simulink model "DC_Motor_Load_PID_tuning_unit_response"  (R2015a)
settings: Solver=ode45  StartTime=0.0  StopTime=10.0  RelTol=1e-3
values from neighbouring files (symbols this model uses):
  BL = B_roller + B_material    (= 0)    [dc_motor_show_data_last.m]    (also in dc_motor_show_data_last_pos.m)
  Bm = 0.0158    [dc_motor_show_data_last.m]    (also in dc_motor_show_data_last_pos.m = 0.00093)
  JL = J_roller + J_material    (= 0.000102958)    [dc_motor_show_data_last.m]    (also in dc_motor_show_data_last_pos.m)
  Jm = 0.00252    [dc_motor_show_data_last.m]    (also in dc_motor_show_data_last_pos.m = 5.26e-05)
  Kd = Kp*Td    (= 8.33268608414)    [ZIEGLER_NICHOLCUS_METHOD_tuning_pid.m]    (also in dc_motor_show_data.m = 0.0189; dc_motor_show_data_PID_range_errors_show.m = 0.09; dc_motor_show_data_PID_range_response.m = 0.09; dc_motor_show_data_PID_test_ST.m = 0.09)
  Ke = 0.1    [DC_MOTOR.m]    (also in ZIEGLER_NICHOLCUS_METHOD_tuning_pid.m = 0.57; dc_motor_show_data.m = 0.57; dc_motor_show_data_PID_range_errors_show.m; dc_motor_show_data_PID_range_response.m)
  Ki = Kp/Ti    (= 21.5184713376)    [ZIEGLER_NICHOLCUS_METHOD_tuning_pid.m]    (also in dc_motor_show_data.m = 39.9; dc_motor_show_data_PID_range_errors_show.m = 2.98; dc_motor_show_data_PID_range_response.m = 2.98; dc_motor_show_data_PID_test_ST.m = 2.98)
  Kp = 0.2*K_cr    (= 16.4)    [ZIEGLER_NICHOLCUS_METHOD_tuning_pid.m]    (also in dc_motor_show_data.m = 2.1398; dc_motor_show_data_PID_range_errors_show.m = 1.25; dc_motor_show_data_PID_range_response.m = 1.25; dc_motor_show_data_PID_test_ST.m = 1.25)
  Kt = 0.2    [DC_MOTOR.m]    (also in ZIEGLER_NICHOLCUS_METHOD_tuning_pid.m = 0.259; dc_motor_show_data.m = 0.259; dc_motor_show_data_PID_range_errors_show.m; dc_motor_show_data_PID_range_response.m)
  La = 0.143    [dc_motor_show_data_last.m]    (also in dc_motor_show_data_last_pos.m = 0.0006)
  Ra = 9.375    [dc_motor_show_data_last.m]    (also in dc_motor_show_data_last_pos.m)
  TL = 0.0017    [dc_motor_show_data_last.m]    (also in dc_motor_show_data_last_pos.m)
settings Model: Creator=Alfa maSR  LastModifiedBy=Alfa maSR

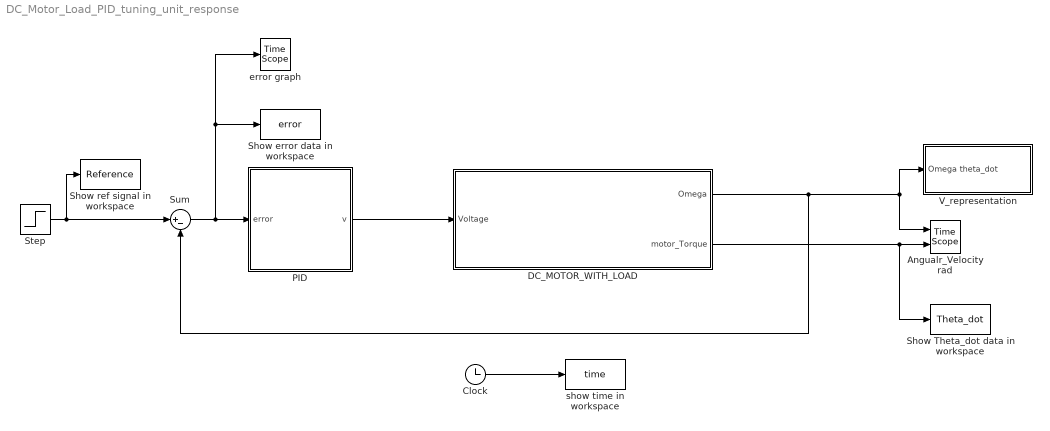
== system DC_Motor_Load_PID_tuning_unit_response ==
  Angualr_Velocity rad : TimeScope  DefaultConfigurationName=spbscopes.TimeScopeBlockCfg  NumInputPorts=2
  Clock : Clock
  DC_MOTOR_WITH_LOAD : Subsystem
  PID : Subsystem
  Show Theta_dot data in workspace : ToWorkspace  VariableName=Theta_dot  SaveFormat=Timeseries  SampleTime=-1
  Show error data in workspace : ToWorkspace  VariableName=error  SaveFormat=Timeseries  SampleTime=-1
  Show ref signal in workspace : ToWorkspace  VariableName=Reference  SaveFormat=Timeseries  SampleTime=-1
  Step : Step  SampleTime=0
  Sum : Sum  Inputs=|+-
  V_representation : Subsystem
  error graph : TimeScope  DefaultConfigurationName=spbscopes.TimeScopeBlockCfg
  show time in workspace : ToWorkspace  VariableName=time  SaveFormat=Timeseries  SampleTime=-1
  wires:
  DC_MOTOR_WITH_LOAD/1(Omega) -> Sum/2, V_representation/1(Omega theta_dot), Angualr_Velocity rad/1
  DC_MOTOR_WITH_LOAD/2(motor_Torque) -> Show Theta_dot data in workspace/1, Angualr_Velocity rad/2
  PID/1(v) -> DC_MOTOR_WITH_LOAD/1(Voltage)
  Clock/1 -> show time in workspace/1
  Step/1 -> Sum/1, Show ref signal in workspace/1
  Sum/1 -> Show error data in workspace/1, error graph/1, PID/1(error)

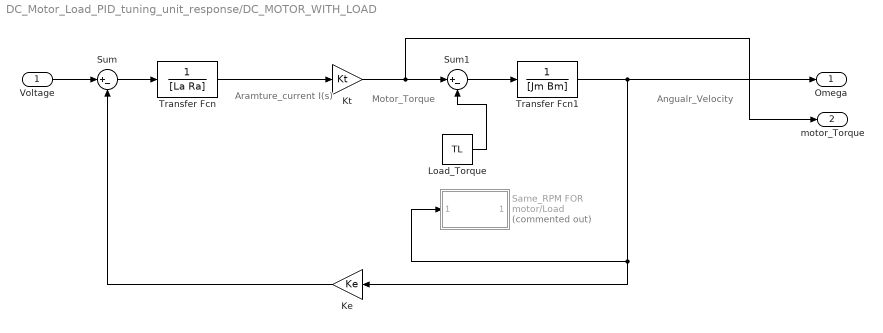
== system DC_Motor_Load_PID_tuning_unit_response/DC_MOTOR_WITH_LOAD ==
  note: Angualr_Velocity
  note: Motor_Torque
  note: Aramture_current
      |           I(s)
  Voltage : Inport
  Ke : Gain  Gain=Ke
  Kt : Gain  Gain=Kt
  Load_Torque : Constant  Value=TL
  Same_RPM FOR motor/Load : Subsystem  Commented=on
  Sum : Sum  Inputs=|+-
  Sum1 : Sum  Inputs=|+-
  Transfer Fcn : TransferFcn  Denominator=[La Ra]
  Transfer Fcn1 : TransferFcn  Denominator=[Jm Bm]
  Omega : Outport
  motor_Torque : Outport  Port=2
  wires:
  Ke/1 -> Sum/2
  Sum1/1 -> Transfer Fcn1/1
  Load_Torque/1 -> Sum1/2
  Sum/1 -> Transfer Fcn/1
  Transfer Fcn/1 -> Kt/1
  Kt/1 -> motor_Torque/1, Sum1/1
  Transfer Fcn1/1 -> Omega/1, Same_RPM FOR motor/Load/1(Omega/ rad/s), Ke/1
  Voltage/1 -> Sum/1

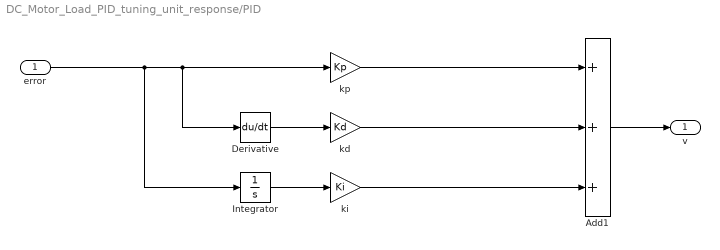
== system DC_Motor_Load_PID_tuning_unit_response/PID ==
  error : Inport
  Add1 : Sum  Inputs=+++
  Derivative : Derivative
  Integrator : Integrator
  kd : Gain  Gain=Kd
  ki : Gain  Gain=Ki
  kp : Gain  Gain=Kp
  v : Outport
  wires:
  error/1 -> kp/1, Derivative/1, Integrator/1
  Add1/1 -> v/1
  ki/1 -> Add1/3
  Integrator/1 -> ki/1
  kp/1 -> Add1/1
  kd/1 -> Add1/2
  Derivative/1 -> kd/1

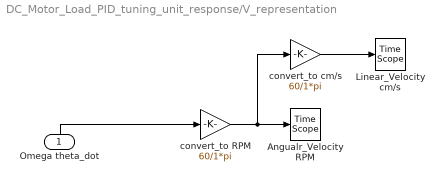
== system DC_Motor_Load_PID_tuning_unit_response/V_representation ==
  Omega theta_dot : Inport
  Angualr_Velocity RPM : TimeScope  DefaultConfigurationName=spbscopes.TimeScopeBlockCfg
  Linear_Velocity cm/s : TimeScope  DefaultConfigurationName=spbscopes.TimeScopeBlockCfg
  convert_to RPM : Gain  Gain=60/1*pi
  convert_to cm/s : Gain  Gain=60/1*pi
  wires:
  Omega theta_dot/1 -> convert_to RPM/1
  convert_to RPM/1 -> Angualr_Velocity RPM/1, convert_to cm/s/1
  convert_to cm/s/1 -> Linear_Velocity cm/s/1

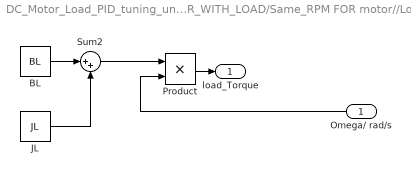
== system DC_Motor_Load_PID_tuning_unit_response/DC_MOTOR_WITH_LOAD/Same_RPM FOR motor//Load ==
  Omega/ rad/s : Inport
  BL : Constant  Value=BL
  JL : Constant  Value=JL
  Product : Product
  Sum2 : Sum  Inputs=|++
  load_Torque : Outport
  wires:
  JL/1 -> Sum2/2
  Omega/ rad/s/1 -> Product/2
  Product/1 -> load_Torque/1
  BL/1 -> Sum2/1
  Sum2/1 -> Product/1
